simulink model "sim_measure_and_Control_WORKS_slidercontrol"  (R2023b)
settings: Solver=FixedStepAuto  StartTime=0.0  StopTime=inf  RelTol=1e-3  EnableMultiTasking=on
libraries: simulink x16, arduinolib x15
settings Model: SimulationMode=external  ExtModeTrigDuration=2  Creator=agraw156  LastModifiedBy=agraw156
settings OptimizationCC: EnhancedBackFolding=on  PassReuseOutputArgsAs=Individual arguments  ZeroExternalMemoryAtStartup=off  ZeroInternalMemoryAtStartup=off  MaxStackSize=64  OptimizeBlockOrder=speed  DifferentSizesBufferReuse=on  OptimizationCustomize=off  EfficientTunableParamExpr=on
settings DebuggingCC: ParameterTunabilityLossMsg=error
settings HardwareCC: ProdBitPerInt=16  ProdBitPerPointer=16  ProdBitPerSizeT=16  ProdBitPerPtrDiffT=16  ProdLargestAtomicFloat=None  ProdWordSize=8  ProdHWDeviceType=Atmel->AVR
settings SFSimCC: MATLABDynamicMemAlloc=off
settings RTWCC: Description=Embedded Coder  SystemTargetFile=ert.tlc  HardwareBoard=Arduino Mega 2560  TemplateMakefile=ert_default_tmf  Toolchain=Arduino AVR  BuildConfiguration=Faster Runs
settings CodeAppCC: ForceParamTrailComments=on  IgnoreCustomStorageClasses=off  OperatorAnnotations=on  SimulinkDataObjDesc=on  SFDataObjDesc=on  InsertBlockDesc=on
settings ERTTargetCC: SupportContinuousTime=on  SupportVariableSizeSignals=on  ExtMode=on  ExtModeTransport=3  ExtModeStaticAlloc=on  ExtModeAutomaticAllocSize=off  ExtModeStaticAllocSize=2048  ExtModeMexFile=ext_xcp  ExtModeMexArgs=0 4 921600  ExtModeIntrfLevel=Level2 - Open

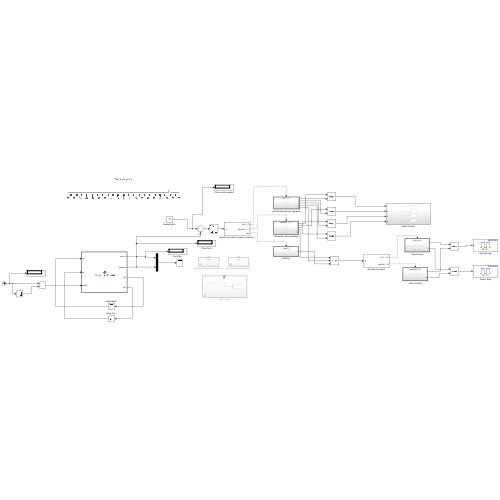
[thumbnail: Simulink's stored preview of the top-level diagram]
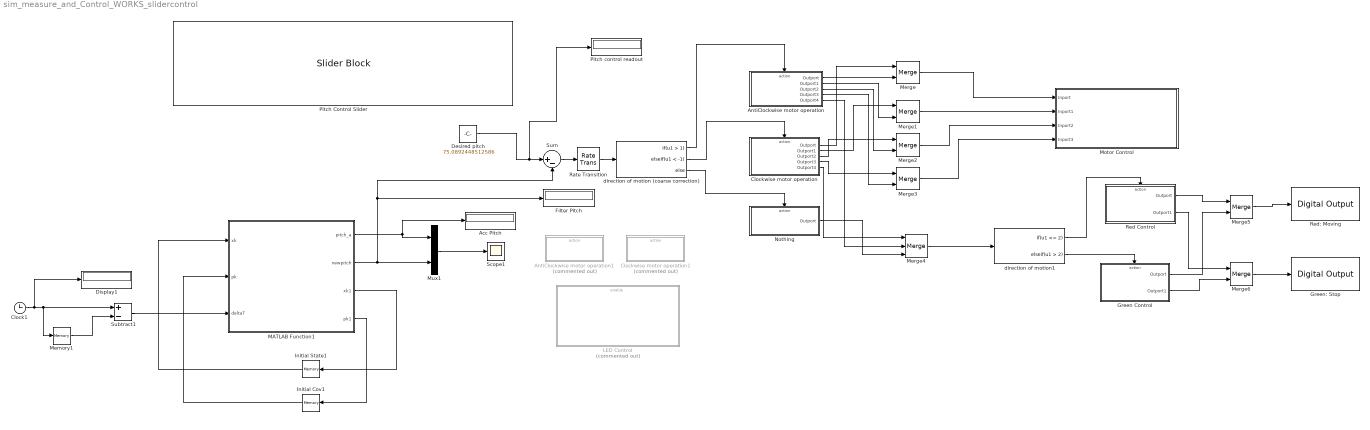
== system sim_measure_and_Control_WORKS_slidercontrol ==
  Acc Pitch : Display
  AntiClockwise motor operation : Subsystem
  AntiClockwise motor operation1 : Subsystem  Commented=on
  Clock1 : Clock
  Clockwise motor operation : Subsystem
  Clockwise motor operation1 : Subsystem  Commented=on
  Desired pitch : Constant  Value=75.0892448512586
  Display1 : Display
  Filter Pitch : Display
  Green Control : Subsystem
  Green: Stop : arduinolib/Digital Output  pinNumber=13  Direction=output  blockPlatform=arduino
  Initial Cov1 : Memory  InitialCondition=[0.5 0; 0 0.01]
  Initial State1 : Memory  InitialCondition=[0;0]
  LED Control : Subsystem  Commented=on
  MATLAB Function1 : MATLAB Function  TreatAsAtomicUnit=on
  Memory1 : Memory
  Merge{,1..3,5..6} (6 alike) : Merge
  Merge4 : Merge  Inputs=3
  Motor Control : Subsystem
  Mux1 : Mux  Inputs=2
  Nothing : Subsystem
  Pitch Control Slider : SliderBlock  ScaleMin=-90  ScaleMax=90  TickInterval=10
  Pitch control readout : Display
  Rate Transition : RateTransition
  Red Control : Subsystem
  Red: Moving : arduinolib/Digital Output  pinNumber=53  Direction=output  blockPlatform=arduino
  Scope1 : Scope
  Subtract1 : Sum  Inputs=+-
  Sum : Sum  Inputs=|+-
  direction of motion (coarse correction) : If  IfExpression=u1 > 1  ElseIfExpressions=u1 < -1
  direction of motion1 : If  IfExpression=u1 <= 2  ElseIfExpressions=u1 > 2  ShowElse=off
  wires:
  MATLAB Function1/3(xk1) -> Initial State1/1
  Initial Cov1/1 -> MATLAB Function1/2(pk)
  MATLAB Function1/2(newpitch) -> Filter Pitch/1, Sum/2, Mux1/2
  Mux1/1 -> Scope1/1
  Initial State1/1 -> MATLAB Function1/1(xk)
  MATLAB Function1/4(pk1) -> Initial Cov1/1
  Memory1/1 -> Subtract1/2
  Clock1/1 -> Subtract1/1, Memory1/1, Display1/1
  Subtract1/1 -> MATLAB Function1/3(deltaT)
  Desired pitch/1 -> Pitch control readout/1, Sum/1
  Sum/1 -> Rate Transition/1
  AntiClockwise motor operation/1(Outport) -> Merge/2
  Clockwise motor operation/1(Outport) -> Merge/1
  Merge/1 -> Motor Control/1(Inport)
  Clockwise motor operation/2(Outport1) -> Merge1/1
  AntiClockwise motor operation/2(Outport1) -> Merge1/2
  Merge1/1 -> Motor Control/2(Inport1)
  Clockwise motor operation/3(Outport2) -> Merge2/1
  AntiClockwise motor operation/3(Outport2) -> Merge2/2
  Merge2/1 -> Motor Control/3(Inport2)
  Merge3/1 -> Motor Control/4(Inport3)
  Clockwise motor operation/4(Outport3) -> Merge3/1
  AntiClockwise motor operation/4(Outport3) -> Merge3/2
  direction of motion (coarse correction)/1 -> AntiClockwise motor operation/Action
  direction of motion (coarse correction)/2 -> Clockwise motor operation/Action
  Rate Transition/1 -> direction of motion (coarse correction)/1
  direction of motion (coarse correction)/3 -> Nothing/Action
  Clockwise motor operation/5(Outport4) -> Merge4/1
  AntiClockwise motor operation/5(Outport4) -> Merge4/2
  Nothing/1(Outport) -> Merge4/3
  Merge4/1 -> direction of motion1/1
  direction of motion1/1 -> Red Control/Action
  direction of motion1/2 -> Green Control/Action
  Red Control/1(Outport) -> Merge5/1
  Green Control/1(Outport) -> Merge5/2
  Merge5/1 -> Red: Moving/1
  Red Control/2(Outport1) -> Merge6/1
  Green Control/2(Outport1) -> Merge6/2
  Merge6/1 -> Green: Stop/1
  MATLAB Function1/1(pitch_a) -> Mux1/1, Acc Pitch/1

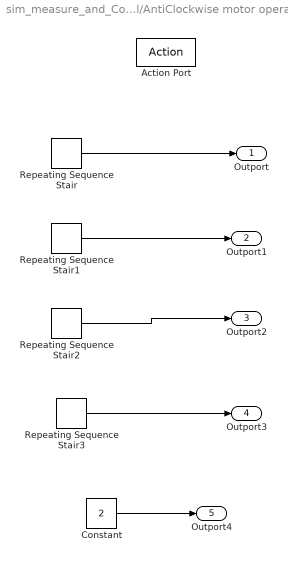
== system sim_measure_and_Control_WORKS_slidercontrol/AntiClockwise motor operation ==
  Action Port : ActionPort  ActionPortLabel=if(u1 > 1)
  Constant : Constant  Value=2
  Repeating Sequence Stair : simulink/Sources/Repeating Sequence Stair  OutValues=[1 0 0 1].'  tsamp=0.002  OutMin=[]  OutMax=[]  OutDataTypeStr=double  OutputDataTypeScalingMode=double  OutDataType=fixdt(0,8)  ConRadixGroup=Best Precision: Vector-wise  OutScaling=2^-12
  Repeating Sequence Stair1 : simulink/Sources/Repeating Sequence Stair  OutValues=[1 1 0 0].'  tsamp=0.002  OutMin=[]  OutMax=[]  OutDataTypeStr=double  OutputDataTypeScalingMode=double  OutDataType=fixdt(0,8)  ConRadixGroup=Best Precision: Vector-wise  OutScaling=2^-12
  Repeating Sequence Stair2 : simulink/Sources/Repeating Sequence Stair  OutValues=[0 1 1 0].'  tsamp=0.002  OutMin=[]  OutMax=[]  OutDataTypeStr=double  OutputDataTypeScalingMode=double  OutDataType=fixdt(0,8)  ConRadixGroup=Best Precision: Vector-wise  OutScaling=2^-12
  Repeating Sequence Stair3 : simulink/Sources/Repeating Sequence Stair  OutValues=[0 0 1 1].'  tsamp=0.002  OutMin=[]  OutMax=[]  OutDataTypeStr=double  OutputDataTypeScalingMode=double  OutDataType=fixdt(0,8)  ConRadixGroup=Best Precision: Vector-wise  OutScaling=2^-12
  Outport : Outport
  Outport1 : Outport  Port=2
  Outport2 : Outport  Port=3
  Outport3 : Outport  Port=4
  Outport4 : Outport  Port=5
  wires:
  Repeating Sequence Stair1/1 -> Outport1/1
  Repeating Sequence Stair2/1 -> Outport2/1
  Repeating Sequence Stair/1 -> Outport/1
  Repeating Sequence Stair3/1 -> Outport3/1
  Constant/1 -> Outport4/1

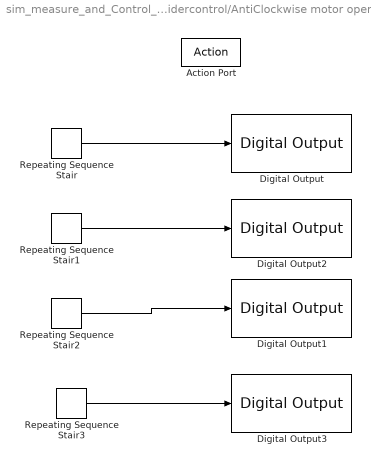
== system sim_measure_and_Control_WORKS_slidercontrol/AntiClockwise motor operation1 ==
  Action Port : ActionPort
  Digital Output : arduinolib/Digital Output  pinNumber=2  Direction=output  blockPlatform=arduino
  Digital Output1 : arduinolib/Digital Output  pinNumber=4  Direction=output  blockPlatform=arduino
  Digital Output2 : arduinolib/Digital Output  pinNumber=3  Direction=output  blockPlatform=arduino
  Digital Output3 : arduinolib/Digital Output  pinNumber=5  Direction=output  blockPlatform=arduino
  Repeating Sequence Stair : simulink/Sources/Repeating Sequence Stair  OutValues=[1 0 0 1].'  tsamp=0.002  OutMin=[]  OutMax=[]  OutDataTypeStr=double  OutputDataTypeScalingMode=double  OutDataType=fixdt(0,8)  ConRadixGroup=Best Precision: Vector-wise  OutScaling=2^-12
  Repeating Sequence Stair1 : simulink/Sources/Repeating Sequence Stair  OutValues=[1 1 0 0].'  tsamp=0.002  OutMin=[]  OutMax=[]  OutDataTypeStr=double  OutputDataTypeScalingMode=double  OutDataType=fixdt(0,8)  ConRadixGroup=Best Precision: Vector-wise  OutScaling=2^-12
  Repeating Sequence Stair2 : simulink/Sources/Repeating Sequence Stair  OutValues=[0 1 1 0].'  tsamp=0.002  OutMin=[]  OutMax=[]  OutDataTypeStr=double  OutputDataTypeScalingMode=double  OutDataType=fixdt(0,8)  ConRadixGroup=Best Precision: Vector-wise  OutScaling=2^-12
  Repeating Sequence Stair3 : simulink/Sources/Repeating Sequence Stair  OutValues=[0 0 1 1].'  tsamp=0.002  OutMin=[]  OutMax=[]  OutDataTypeStr=double  OutputDataTypeScalingMode=double  OutDataType=fixdt(0,8)  ConRadixGroup=Best Precision: Vector-wise  OutScaling=2^-12
  wires:
  Repeating Sequence Stair1/1 -> Digital Output2/1
  Repeating Sequence Stair2/1 -> Digital Output1/1
  Repeating Sequence Stair/1 -> Digital Output/1
  Repeating Sequence Stair3/1 -> Digital Output3/1

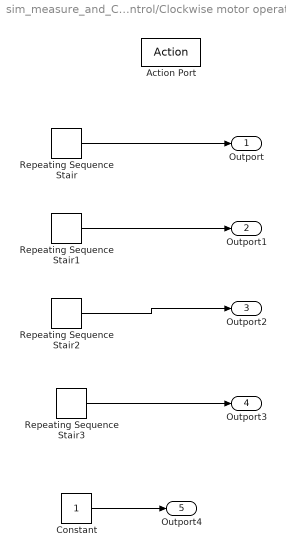
== system sim_measure_and_Control_WORKS_slidercontrol/Clockwise motor operation ==
  Action Port : ActionPort  ActionPortLabel=elseif(u1 < -1)
  Constant : Constant
  Repeating Sequence Stair : simulink/Sources/Repeating Sequence Stair  OutValues=[1 0 0 1].'  tsamp=0.002  OutMin=[]  OutMax=[]  OutDataTypeStr=double  OutputDataTypeScalingMode=double  OutDataType=fixdt(0,8)  ConRadixGroup=Best Precision: Vector-wise  OutScaling=2^-12
  Repeating Sequence Stair1 : simulink/Sources/Repeating Sequence Stair  OutValues=[0 0 1 1].'  tsamp=0.002  OutMin=[]  OutMax=[]  OutDataTypeStr=double  OutputDataTypeScalingMode=double  OutDataType=fixdt(0,8)  ConRadixGroup=Best Precision: Vector-wise  OutScaling=2^-12
  Repeating Sequence Stair2 : simulink/Sources/Repeating Sequence Stair  OutValues=[0 1 1 0].'  tsamp=0.002  OutMin=[]  OutMax=[]  OutDataTypeStr=double  OutputDataTypeScalingMode=double  OutDataType=fixdt(0,8)  ConRadixGroup=Best Precision: Vector-wise  OutScaling=2^-12
  Repeating Sequence Stair3 : simulink/Sources/Repeating Sequence Stair  OutValues=[1 1 0 0].'  tsamp=0.002  OutMin=[]  OutMax=[]  OutDataTypeStr=double  OutputDataTypeScalingMode=double  OutDataType=fixdt(0,8)  ConRadixGroup=Best Precision: Vector-wise  OutScaling=2^-12
  Outport : Outport
  Outport1 : Outport  Port=2
  Outport2 : Outport  Port=3
  Outport3 : Outport  Port=4
  Outport4 : Outport  Port=5
  wires:
  Repeating Sequence Stair3/1 -> Outport3/1
  Repeating Sequence Stair/1 -> Outport/1
  Repeating Sequence Stair2/1 -> Outport2/1
  Repeating Sequence Stair1/1 -> Outport1/1
  Constant/1 -> Outport4/1

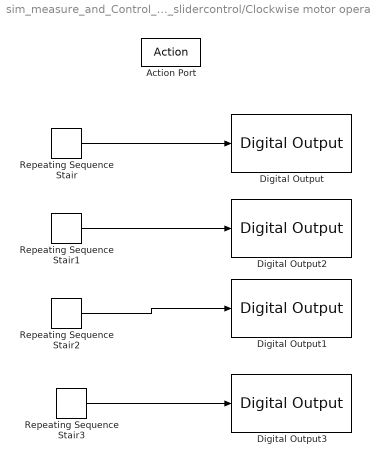
== system sim_measure_and_Control_WORKS_slidercontrol/Clockwise motor operation1 ==
  Action Port : ActionPort
  Digital Output : arduinolib/Digital Output  pinNumber=2  Direction=output  blockPlatform=arduino
  Digital Output1 : arduinolib/Digital Output  pinNumber=4  Direction=output  blockPlatform=arduino
  Digital Output2 : arduinolib/Digital Output  pinNumber=3  Direction=output  blockPlatform=arduino
  Digital Output3 : arduinolib/Digital Output  pinNumber=5  Direction=output  blockPlatform=arduino
  Repeating Sequence Stair : simulink/Sources/Repeating Sequence Stair  OutValues=[1 0 0 1].'  tsamp=0.002  OutMin=[]  OutMax=[]  OutDataTypeStr=double  OutputDataTypeScalingMode=double  OutDataType=fixdt(0,8)  ConRadixGroup=Best Precision: Vector-wise  OutScaling=2^-12
  Repeating Sequence Stair1 : simulink/Sources/Repeating Sequence Stair  OutValues=[0 0 1 1].'  tsamp=0.002  OutMin=[]  OutMax=[]  OutDataTypeStr=double  OutputDataTypeScalingMode=double  OutDataType=fixdt(0,8)  ConRadixGroup=Best Precision: Vector-wise  OutScaling=2^-12
  Repeating Sequence Stair2 : simulink/Sources/Repeating Sequence Stair  OutValues=[0 1 1 0].'  tsamp=0.002  OutMin=[]  OutMax=[]  OutDataTypeStr=double  OutputDataTypeScalingMode=double  OutDataType=fixdt(0,8)  ConRadixGroup=Best Precision: Vector-wise  OutScaling=2^-12
  Repeating Sequence Stair3 : simulink/Sources/Repeating Sequence Stair  OutValues=[1 1 0 0].'  tsamp=0.002  OutMin=[]  OutMax=[]  OutDataTypeStr=double  OutputDataTypeScalingMode=double  OutDataType=fixdt(0,8)  ConRadixGroup=Best Precision: Vector-wise  OutScaling=2^-12
  wires:
  Repeating Sequence Stair3/1 -> Digital Output3/1
  Repeating Sequence Stair/1 -> Digital Output/1
  Repeating Sequence Stair2/1 -> Digital Output1/1
  Repeating Sequence Stair1/1 -> Digital Output2/1

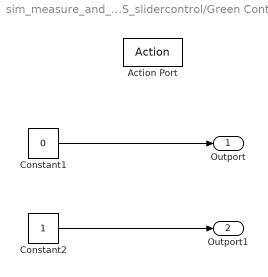
== system sim_measure_and_Control_WORKS_slidercontrol/Green Control ==
  Action Port : ActionPort  ActionPortLabel=elseif(u1 > 2)
  Constant1 : Constant  Value=0
  Constant2 : Constant
  Outport : Outport
  Outport1 : Outport  Port=2
  wires:
  Constant1/1 -> Outport/1
  Constant2/1 -> Outport1/1

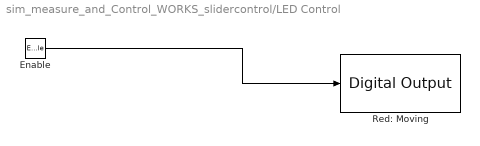
== system sim_measure_and_Control_WORKS_slidercontrol/LED Control ==
  Enable : EnablePort  StatesWhenEnabling=reset  ShowOutputPort=on
  Red: Moving : arduinolib/Digital Output  pinNumber=7  Direction=output  blockPlatform=arduino
  wires:
  Enable/1 -> Red: Moving/1

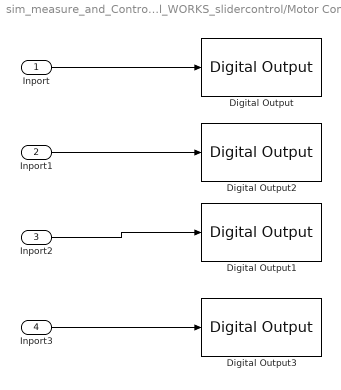
== system sim_measure_and_Control_WORKS_slidercontrol/Motor Control ==
  Inport : Inport
  Inport1 : Inport  Port=2
  Inport2 : Inport  Port=3
  Inport3 : Inport  Port=4
  Digital Output : arduinolib/Digital Output  pinNumber=2  Direction=output  blockPlatform=arduino
  Digital Output1 : arduinolib/Digital Output  pinNumber=4  Direction=output  blockPlatform=arduino
  Digital Output2 : arduinolib/Digital Output  pinNumber=3  Direction=output  blockPlatform=arduino
  Digital Output3 : arduinolib/Digital Output  pinNumber=5  Direction=output  blockPlatform=arduino
  wires:
  Inport1/1 -> Digital Output2/1
  Inport2/1 -> Digital Output1/1
  Inport/1 -> Digital Output/1
  Inport3/1 -> Digital Output3/1

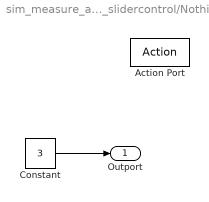
== system sim_measure_and_Control_WORKS_slidercontrol/Nothing ==
  Action Port : ActionPort  ActionPortLabel=else
  Constant : Constant  Value=3
  Outport : Outport
  wires:
  Constant/1 -> Outport/1

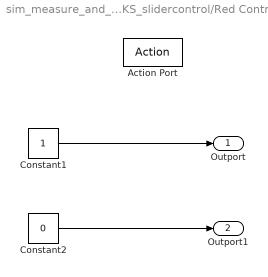
== system sim_measure_and_Control_WORKS_slidercontrol/Red Control ==
  Action Port : ActionPort  ActionPortLabel=if(u1 <= 2)
  Constant1 : Constant
  Constant2 : Constant  Value=0
  Outport : Outport
  Outport1 : Outport  Port=2
  wires:
  Constant2/1 -> Outport1/1
  Constant1/1 -> Outport/1

== matlab function sim_measure_and_Control_WORKS_slidercontrol/MATLAB Function1 ==
  data: pitch_a output; newpitch output; xk1 output; xk input; pk input; deltaT input; pk1 output
function [pitch_a,newpitch,xk1,pk1] = calculate_angle_pitch(xk,pk,deltaT)
% Calculate ypr using acclerometer and gyroscope separately yaw_g, pitch_g, roll_g,

persistent arduinoObj imuObj 

if isempty(arduinoObj)
    arduinoObj = arduino();
end
if isempty(imuObj)
    imuObj = mpu6050(arduinoObj);
end

% Reading data from Arduino 

    [accel,gyro] = read(imuObj);

    ax=accel(1);
    ay=accel(2);
    az=accel(3);
    
    Vx=gyro(1);
    Vy=gyro(2);
    Vz=gyro(3);   


% Kalman filter parameters

%xk = zeros(2,1); % roll angle and drift 
%pk = [0.5 0; 0 0.01]; % Covariance

%K = zeros(2,1); 
phi = [1 -deltaT; 0 1]; % STM (A)
psi = [deltaT ;0]; % Mapping Matrix (B)

R = 0.03; % measurement noise (accelerometer correction to gyro drift)
Q = [0.001 0 ;0 0.003]; % Process noise
H = [1 0]; % observation matrix

pitch_a = atand(ax/sqrt((ay*ay) + (az*az)));

uk = Vy; 
zk = pitch_a; 
% Prediction
    xk1Minus = phi * xk + psi * uk; 
    pk1Minus = phi * pk * phi' + Q*deltaT; 

% Correction
    S = H*pk1Minus*H' + R; % Intermediate term (used in the kalman gain)
    K = pk1Minus*H'*inv(S); % Kalman gain

    y = zk - H*xk1Minus;
    xk1 = xk1Minus + K*y; 
    pk1 = (eye(2) - K*H)*pk1Minus; 
    newpitch = xk(1);    

    % xk = xk1; 
    % pk = pk1; 


end
